simulink model "test_mismatch"  (R2022a)
settings: Solver=VariableStepAuto  StartTime=0.0  StopTime=10.0  RelTol=1e-3
model workspace (MAT data in the model file):
  gfm = 3
  gsm = 2.3
libraries: neuromorphic_blocks x7
settings Model: Creator=chris  LastModifiedBy=chris

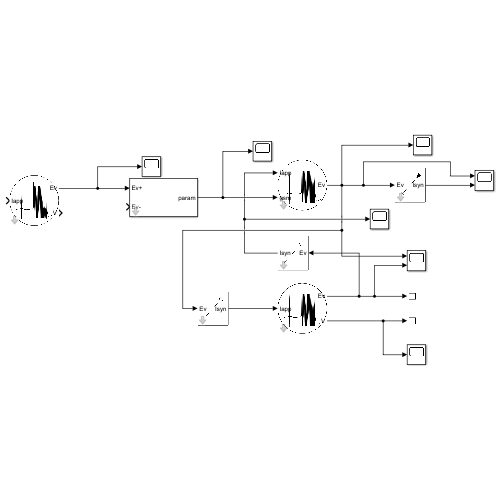
[thumbnail: Simulink's stored preview of the top-level diagram]
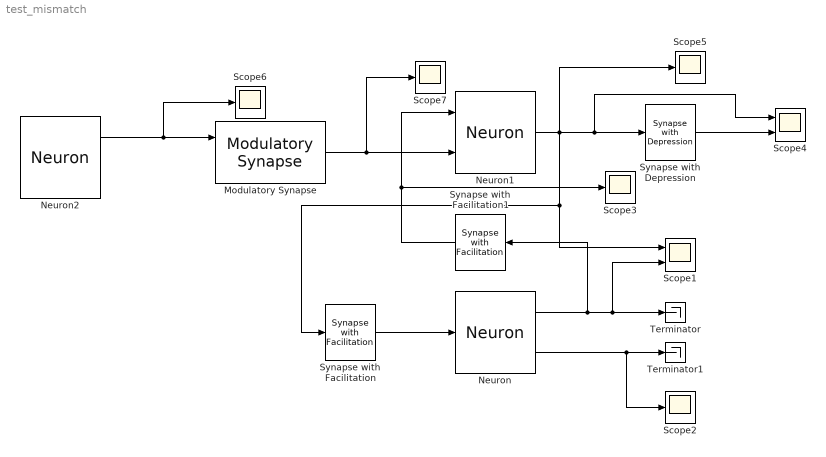
== system test_mismatch ==
  Modulatory Synapse : neuromorphic_blocks/Neural Blocks/Modulatory Synapse  base_val=2.3  gsyn_pos_source=Internal  gsyn_pos=2  gsyn_neg_source=Internal  gsyn_neg=2  timescale=0.004  rel_timescale=1000  input=Events  dsyn_pos=0  dsyn_neg=0  msyn_pos=1  msyn_neg=1
      settings: SourceProductName=Neuromorphic Toolbox
  Neuron : neuromorphic_blocks/Neural Blocks/Neuron  gfm_source=Internal  gfm=3  gsp_source=Internal  gsp=6  gsm_source=Internal  gsm=2.3  gup_source=Internal  gup=5  gum_source=Internal  gum=2  dfm=0  dsp=0.5  dsm=-0.5  dup=-0.5  dum=-1  mfm=1  msp=1  msm=1  mup=1  mum=1  timescale=0.004  rel_membrane=0.1  rel_fast=0.1  rel_slow=4  rel_ultraslow=200  Iapp_base=0.11  V0=-1.2  tresh=0  output=Both
      settings: SourceProductName=Neuromorphic Toolbox
  Neuron1 : neuromorphic_blocks/Neural Blocks/Neuron  gfm_source=Internal  gfm=3  gsp_source=Internal  gsp=6  gsm_source=External  gsm=2.3  gup_source=Internal  gup=5  gum_source=Internal  gum=2  dfm=0  dsp=0.5  dsm=-0.5  dup=-0.5  dum=-1  mfm=1  msp=1  msm=1  mup=1  mum=1  timescale=0.004  rel_membrane=0.1  rel_fast=0.1  rel_slow=4  rel_ultraslow=200  Iapp_base=0.1  V0=-1.2  tresh=0  output=Events
      settings: SourceProductName=Neuromorphic Toolbox
  Neuron2 : neuromorphic_blocks/Neural Blocks/Neuron  gfm_source=Internal  gfm=2  gsp_source=Internal  gsp=5  gsm_source=Internal  gsm=1  gup_source=Internal  gup=1  gum_source=Internal  gum=0  dfm=0  dsp=0.5  dsm=-0.5  dup=-0.5  dum=-1  mfm=1  msp=1  msm=1  mup=1  mum=1  timescale=0.004  rel_membrane=0.1  rel_fast=0.1  rel_slow=4  rel_ultraslow=200  Iapp_base=0.5  V0=-1.2  tresh=0  output=Both
      settings: SourceProductName=Neuromorphic Toolbox
  Scope1 : Scope  NumInputPorts=2
  Scope{2..3,5..7} (5 alike) : Scope
  Scope4 : Scope  NumInputPorts=2
  Synapse with Depression : neuromorphic_blocks/Neural Blocks/Synapse with Depression  gsyn_source=Internal  gsyn=2  dsyn=10  msyn=50  dsyn_dep=-10  msyn_dep=50  timescale=0.004  rel_timescale=100  input=Events  gsyn_in=0  dsyn_in=0  msyn_in=1
      settings: SourceProductName=Neuromorphic Toolbox
  Synapse with Facilitation : neuromorphic_blocks/Neural Blocks/Synapse with Facilitation  gsyn_source=Internal  gsyn=-1  dsyn=2  msyn=5  timescale=0.004  rel_timescale=10  input=Events  gsyn_in=0  dsyn_in=0  msyn_in=1
      settings: SourceProductName=Neuromorphic Toolbox
  Synapse with Facilitation1 : neuromorphic_blocks/Neural Blocks/Synapse with Facilitation  gsyn_source=Internal  gsyn=-1  dsyn=2  msyn=5  timescale=0.004  rel_timescale=10  input=Events  gsyn_in=0  dsyn_in=0  msyn_in=1
      settings: SourceProductName=Neuromorphic Toolbox
  Terminator : Terminator
  Terminator1 : Terminator
  wires:
  Neuron/1 -> Synapse with Facilitation1/1, Scope1/2, Terminator/1
  Neuron/2 -> Scope2/1, Terminator1/1
  Synapse with Facilitation/1 -> Neuron/1
  Neuron1/1 -> Scope1/1, Synapse with Facilitation/1, Scope5/1, Scope4/1, Synapse with Depression/1
  Synapse with Facilitation1/1 -> Neuron1/1, Scope3/1
  Synapse with Depression/1 -> Scope4/2
  Modulatory Synapse/1 -> Scope7/1, Neuron1/2
  Neuron2/1 -> Scope6/1, Modulatory Synapse/1
